simulink model "tether_model"  (R2021b)
settings: Solver=VariableStepAuto  StartTime=0.0  StopTime=1.5*3600  RelTol=1e-3
model workspace (MAT data in the model file):
  At = 7.85398163397e-07
  Is = 1800595238.1
  L = 5000
  a = 7378
  ecc = 0.001
  gamma = 0.00015
  m = 350
  mu_m = 8.22e+22
  p = 0.0031
undefined symbols (not defined in the file): me
settings Model: Creator=woo  LastModifiedBy=woo

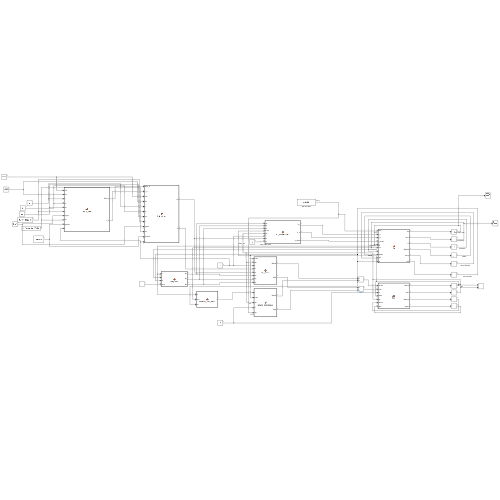
[thumbnail: Simulink's stored preview of the top-level diagram]
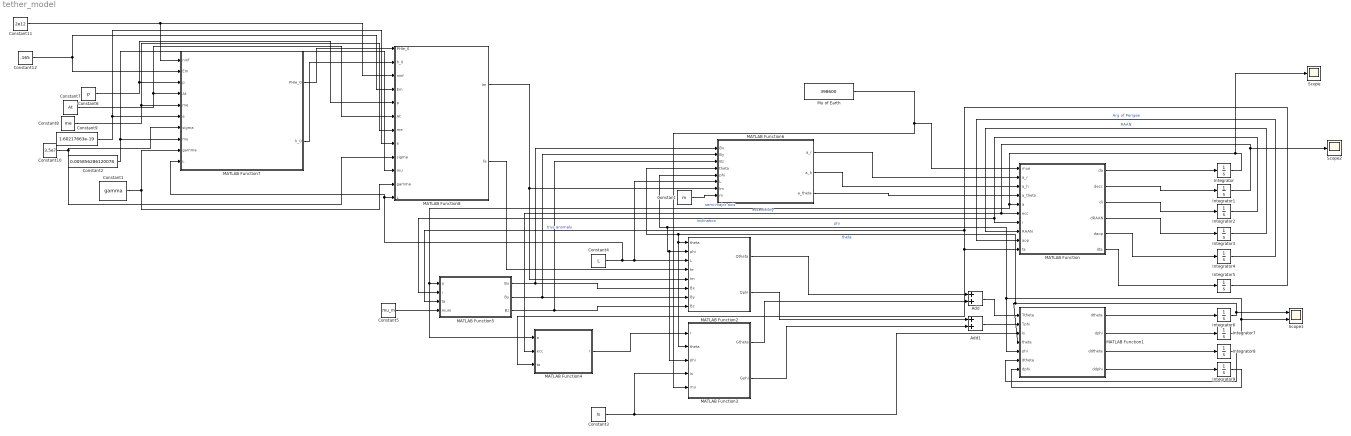
== system tether_model ==
  Add : Sum
  Add1 : Sum
  Constant : Constant  Value=m
  Constant1 : Constant  Value=gamma
  Constant10 : Constant  Value=3.5e7
  Constant11 : Constant  Value=2e12
  Constant12 : Constant  Value=.165
  Constant2 : Constant  Value=0.005856286120078
  Constant3 : Constant  Value=Is
  Constant4 : Constant  Value=L
  Constant5 : Constant  Value=mu_m
  Constant6 : Constant  Value=p
  Constant7 : Constant  Value=At
  Constant8 : Constant  Value=me
  Constant9 : Constant  Value=1.60217663e-19
  Integrator : Integrator  InitialCondition=a
  Integrator1 : Integrator  InitialCondition=ecc
  Integrator2 : Integrator  InitialCondition=deg2rad(25)
  Integrator{3..5,8..9} (5 alike) : Integrator
  Integrator6 : Integrator  InitialCondition=0.1
  Integrator7 : Integrator  InitialCondition=0.1
  MATLAB Function : MATLAB Function  TreatAsAtomicUnit=on
  MATLAB Function1 : MATLAB Function  TreatAsAtomicUnit=on
  MATLAB Function2 : MATLAB Function  TreatAsAtomicUnit=on
  MATLAB Function3 : MATLAB Function  TreatAsAtomicUnit=on
  MATLAB Function4 : MATLAB Function  TreatAsAtomicUnit=on
  MATLAB Function5 : MATLAB Function  TreatAsAtomicUnit=on
  MATLAB Function6 : MATLAB Function  TreatAsAtomicUnit=on
  MATLAB Function7 : MATLAB Function  TreatAsAtomicUnit=on
      settings: RTWSystemCode=Nonreusable function
  MATLAB Function8 : MATLAB Function  TreatAsAtomicUnit=on
  Mu of Earth : Constant  Value=398600  VectorParams1D=off
  Scope : Scope
  Scope1 : Scope  NumInputPorts=2
  Scope2 : Scope
  wires:
  MATLAB Function/1(da) -> Integrator/1
  Integrator/1 -> Scope/1, MATLAB Function4/1(a), MATLAB Function5/1(a), MATLAB Function/5(a)  "semi-major axis"
  MATLAB Function6/3(a_theta) -> MATLAB Function/4(a_theta)
  MATLAB Function6/2(a_h) -> MATLAB Function/3(a_h)
  MATLAB Function6/1(a_r) -> MATLAB Function/2(a_r)
  MATLAB Function/2(decc) -> Integrator1/1
  Integrator1/1 -> Scope2/1, MATLAB Function4/2(ecc), MATLAB Function/6(ecc)  "eccentricity"
  MATLAB Function/3(di) -> Integrator2/1
  Integrator2/1 -> MATLAB Function5/2(i), MATLAB Function/7(i)  "inclination"
  MATLAB Function/4(dRAAN) -> Integrator3/1
  Integrator3/1 -> MATLAB Function/8(RAAN)  "RAAN"
  MATLAB Function/5(daop) -> Integrator4/1
  Integrator4/1 -> MATLAB Function/9(aop)  "Arg of Perigee"
  Integrator5/1 -> MATLAB Function4/3(ta), MATLAB Function/10(ta), MATLAB Function5/3(ta)  "true anomaly"
  MATLAB Function/6(dta) -> Integrator5/1
  Mu of Earth/1 -> MATLAB Function3/5(mu), MATLAB Function/1(mue)
  MATLAB Function1/1(dtheta) -> Integrator6/1
  MATLAB Function1/2(dphi) -> Integrator7/1
  MATLAB Function1/4(ddphi) -> Integrator9/1
  MATLAB Function1/3(ddtheta) -> Integrator8/1
  Integrator9/1 -> MATLAB Function1/7("dphi ")
  Integrator8/1 -> MATLAB Function1/6("dtheta ")
  Integrator7/1 -> MATLAB Function1/5(phi), MATLAB Function3/3(phi), MATLAB Function2/2(phi), MATLAB Function6/5(phi), Scope1/2  "phi"
  Integrator6/1 -> MATLAB Function3/2(theta), MATLAB Function2/1(theta), MATLAB Function6/4(theta), MATLAB Function1/4(theta), Scope1/1  "theta"
  Constant3/1 -> MATLAB Function3/4(Is), MATLAB Function1/3(Is)
  MATLAB Function2/1(Qtheta) -> Add/1
  MATLAB Function3/1(Gtheta) -> Add/2
  Add/1 -> MATLAB Function1/1(Ttheta)
  Add1/1 -> MATLAB Function1/2(Tphi)
  MATLAB Function2/2(Qphi) -> Add1/1
  MATLAB Function3/2(Gphi) -> Add1/2
  Constant4/1 -> MATLAB Function7/10(L), MATLAB Function8/12(L), MATLAB Function6/6(L), MATLAB Function2/3(L)
  MATLAB Function5/1(Bx) -> MATLAB Function6/1(Bx), MATLAB Function2/6(Bx)
  MATLAB Function5/2(By) -> MATLAB Function6/2(By), MATLAB Function2/7(By)
  MATLAB Function5/3(Bz) -> MATLAB Function6/3(Bz), MATLAB Function2/8(Bz)
  Constant5/1 -> MATLAB Function5/4(mum)
  MATLAB Function4/1(r) -> MATLAB Function3/1(r)
  Constant/1 -> MATLAB Function6/8(m)
  MATLAB Function7/1(PHIe_0) -> MATLAB Function8/1(PHIe_0)
  MATLAB Function7/2(h_0) -> MATLAB Function8/2(h_0)
  Constant1/1 -> MATLAB Function7/9(gamma), MATLAB Function8/11(gamma)
  Constant6/1 -> MATLAB Function8/5(p), MATLAB Function7/3(p)
  Constant7/1 -> MATLAB Function8/6(At), MATLAB Function7/4(At)
  Constant2/1 -> MATLAB Function8/10(mu), MATLAB Function7/8(mu)
  Constant8/1 -> MATLAB Function8/7(me), MATLAB Function7/5(me)
  Constant9/1 -> MATLAB Function8/8(e), MATLAB Function7/6(e)
  Constant10/1 -> MATLAB Function8/9(sigma), MATLAB Function7/7(sigma)
  Constant12/1 -> MATLAB Function8/4(Em), MATLAB Function7/2(Em)
  Constant11/1 -> MATLAB Function8/3(ninf), MATLAB Function7/1(ninf)
  MATLAB Function8/1(Im) -> MATLAB Function2/5(Im), MATLAB Function6/7(Im)
  MATLAB Function8/2(fe) -> MATLAB Function2/4(fe)

== matlab function tether_model/MATLAB Function5 ==
  data: a input; Bx output; i input; ta input; mum input; By output; Bz output
function [Bx, By, Bz] = MagField(a, i, ta, mum)
    % Earthrs magnetic field vector in the Orbital Frame of SBET paper
    % SI units output

    % Define variables
    a = COES(1);
    i = COES(3);
    ta = COES(6);
    
%     Bo = 3.12e-5;
%     Bo_over_R3 = Bo/((p/(1+e*cos(ta)))/6378)^3;
    constant = mum/((a*1e3)^3);

    Bx = -2*constant*sin(i)*sin(ta);
    By = -constant*cos(i);
    Bz = constant*sin(i)*cos(ta);

== matlab function tether_model/MATLAB Function6 ==
  data: Bx input; a_r output; By input; Bz input; theta input; phi input; L input; Im input; m input; a_h output; a_theta output
function [a_r, a_h, a_theta] = edt_accelerations(Bx, By, Bz, theta, phi, L, Im, m)
    uhat = [cos(phi)*cos(theta), -sin(phi), cos(phi)*sin(theta)];
    f_orbital = Im*L*cross(uhat, [Bx, By, Bz]);
    a_orbital = f_orbital/m*1e-3'; % force to acceleraction in m to km
    a_r = a_orbital(1);
    a_h = a_orbital(2);
    a_theta = a_orbital(3);

== matlab function tether_model/MATLAB Function7 ==
  data: ninf input; Em input; p input; PHIe_0 output; At input; me input; e input; sigma input; mu input; gamma input; L input; h_0 output
function [PHIe_0, h_0] = solve_bvp(ninf, Em, p, At, me, e, sigma, mu, gamma, L)
    net = load("nna_L4N16_1e2_1e2_100_5km_5mm.mat");
    output = net.net([1;1;1;Em/100;ninf/2e12]);
    PHIe_0 = output(3)*1e5;
    h_0 = output(1)*1e3;
% function [PHIe_0, h_0] = solve_bvp(ninf, Em, p, At, me, e, sigma, mu, gamma, L)
%     parameters = [p, At, me, Em, e, sigma, ninf, mu, gamma];
%     I_B_0 = 1;
%     h0_0 = L/10;
%     s0 = [1;I_B_0;h0_0];
%     opts = optimoptions( 'fsolve' , 'Display' , 'off'  , 'FunctionTolerance' , 1e-8 ,...
%         'StepTolerance' , 1e-8 , 'OptimalityTolerance' , 1e-8 , ...
%         'Algorithm' , 'levenberg-marquardt') ; 
%     [ s0s , F ] = fsolve( @(s)TetherSolveFun(s,parameters,L) , s0 , opts) ;
%     PHIe_0 = s0s(1); 
%     I_B = s0s(2);
%     h_0 = s0s(3);
% 
% 
% end
% 
% 
%     function F = TetherSolveFun(s0, parameters, L) % boundary conditions  
%         p = parameters(1); %perimeter in meters
%         At = parameters(2);
%         me = parameters(3); % mass of electron
%         Em = parameters(4); % Induced electric field; dot(cross(v, B), u)
%         e = parameters(5); % electron charge
%         sigma = parameters(6); % from paper
%         ninf = parameters(7); % ionospheric plasma density 
%         mu = parameters(8); % apparently for atomic oxygen
%         gamma = parameters(9);
%     
%         Ie_0 = 0;
%         PHIe_0 = s0(1); 
%         I_B = s0(2);
%         h0 = s0(3);
%         state0 = [Ie_0, PHIe_0];
%         h_span1 = [0, h0] ;
%         h_span2 = [h0, L] ;
%         opts = odeset( 'RelTol' , 1e-8 , 'AbsTol' , 1e-8 ) ;
%         [t1, s1] = ode45( @bvp_ode_low, h_span1, state0, opts) ;
%         sB = s1(end,:);
%         [t2, s2] = ode45( @bvp_ode_high, h_span2, sB, opts) ;
%         sf = s2(end,:);
%         % [ie, phie]
%     
%         F(1) = sB(1)-I_B; % Ie = max current = I_B, at B
%         F(2) = sB(2); % PHIe = 0 at B
%         F(3) = sf(1)*100; % Ie = 0, I_B, at B
%         F(4) = sum(abs(s1(:,2))-s1(:,2));
%     
%     
%         function dstate = bvp_ode_low(h,state) % equation being solved
%             Ie = state(1);
%             PHIe = state(2);
%               
%             dstate = zeros(2,1);
%             dstate(1) = e*ninf*p/pi*sqrt((2*e/me)*abs(PHIe));
%             dstate(2) = Ie/(sigma*At)-Em;
%         end
%     
%         function dstate = bvp_ode_high(h,state) % equation being solved
%             Ie = state(1);
%             PHIe = state(2);
%         
%             dstate = zeros(2,1);
%             dstate(1) = -e*ninf*p/pi*sqrt((2*e/me)*abs(PHIe))*mu*(1+gamma*abs(PHIe));
%             dstate(2) = Ie/(sigma*At)-Em;
%         end
%     end

== matlab function tether_model/MATLAB Function8 ==
  data: PHIe_0 input; h_0 input; ninf input; Em input; p input; At input; me input; e input; sigma input; mu input; gamma input; L input; Im output; fe output
function [Im, fe] = find_current(PHIe_0, h_0, ninf, Em, p, At, me, e, sigma, mu, gamma, L)
    h_span = [0, L];
    parameters = [p, At, me, Em, e, sigma, ninf, mu, gamma, h_0];
    opts = odeset( 'RelTol' , 1e-8 , 'AbsTol' , 1e-8 ) ;
    [h, s] = ode45( @current_distribution_diffe, h_span, [0, PHIe_0], opts, parameters) ;
    J1 = 0;
    Iint = 0;
    fe_right = 0;
    for ii = 2:length(h)
        J1 = J1 + ((h_G-h(ii))*(s(ii,1))+(h_G-h(ii-1))*(s(ii-1,1)))/2*(h(ii)-h(ii-1));
        Iint = Iint + (s(ii,1)+s(ii-1,1))/2*(h(ii)-h(ii-1));
        fe_right = fe_right + (h(ii)*s(ii,1) + h(ii-1)*s(ii-1,1))/2 * (h(ii)-h(ii-1));
    end
    epsilon = (J1/Is)*mum/mue_si;
    Im = Iint/L;
    fe = fe_right/(L^2*Im);

== matlab function tether_model/MATLAB Function1 ==
  data: dtheta output; dphi output; Ttheta input; ddtheta output; Tphi input; Is input; theta input; phi input; dtheta input; dphi input; ddphi output
function [dtheta, dphi, ddtheta, ddphi] = fcn(Ttheta, Tphi, Is, theta, phi, dtheta, dphi)
    ddtheta = T(2)/Is;
    ddphi = T(3)/Is;

== matlab function tether_model/MATLAB Function ==
  data: mue input; a_r input; da output; a_h input; a_theta input; a input; ecc input; i input; RAAN input; aop input; ta input; decc output; di output; dRAAN output; daop output; dta output
function [da, decc, di, dRAAN, daop, dta]  = VoP(mue, a_r, a_h, a_theta, a, ecc, i, RAAN, aop, ta)
%     a = state(1);
%     ecc = state(2);
%     i = state(3);
%     RAAN = state(4);
%     aop = state(5);
%     ta = state(6);

    p = a*(1-ecc^2);
    h = sqrt(mue*p);
    r = p/(1+ecc*cos(ta));
    n = sqrt(mue/a^3);
    u = aop + ta;

    da = (2/(n*sqrt(1-ecc^2)))*(ecc*sin(ta)*a_r + (p/r)*a_theta);
    decc = (sqrt(1-ecc^2)/(n*a))*(sin(ta)*a_r + ...
        (cos(ta)+(ecc+cos(ta))/(1+ecc*cos(ta)))*a_theta);
    di = (r*cos(u)/(n*a^2*sqrt(1-ecc^2)))*a_h;
    dRAAN = (r*sin(u)/(n*a^2*sqrt(1-ecc^2)*sin(i)))*a_h;
    daop = (sqrt(1-ecc^2)/(n*a*ecc))*(-cos(ta)*a_r + ...
        sin(ta)*(1+r/p)*a_theta) - (r*cot(i)*sin(u)/h)*a_r;
    dta = h/r^2 + (1/(ecc*h))*(p*cos(ta)*a_r - (p+r)*sin(ta)*a_theta);

== matlab function tether_model/MATLAB Function2 ==
  data: theta input; Qtheta output; phi input; L input; fe input; Im input; Bx input; By input; Bz input; Qphi output
function [Qtheta, Qphi] = edt_torque(theta, phi, L, fe, Im, Bx, By, Bz)
    % x is towards zenith
    % y is -h, rotation is in-plane or theta
    % z is along track, rotation is out-of-plane or phi

    Qtheta = fe*Im*L^2*cos(phi)*(sin(phi)*(Bx*cos(theta)+Bz*sin(theta))+By*cos(phi));
    Qphi = -fe*Im*L^2*(Bx*sin(theta)-Bz*cos(theta));

== matlab function tether_model/MATLAB Function3 ==
  data: r input; Gtheta output; theta input; phi input; Is input; mu input; Gphi output
function [Gtheta, Gphi] = gravity_grad_torque(r, theta, phi, Is, mu)
    % Finds the gravity gradient torque effecting the tether
    % x is towards zenith
    % y is -h, rotation is in-plane or theta
    % z is along track, rotation is out-of-plane or phi
    inertia = [0, 0, 0; 0, Is, 0; 0, 0, Is];

    % Dynamics from "Spacecraft Dynamics and Control"
    u1 = [cos(phi)*cos(theta); -sin(phi); cos(phi)*sin(theta)];
    u2 = [-sin(theta); 0; cos(theta)];
    u3 = [-sin(phi)*cos(theta); -cos(phi); -sin(phi)*sin(theta)];
    tether_rotation = [u1, u2, u3];
    rb = tether_rotation*[r;0;0];

    % transform inertia into eci
    rbcross = [0, -rb(3), rb(2);
                rb(3), 0, -rb(1);
                -rb(2), rb(2), 0];
    Tgg = ((3*mu/r^5 * rbcross*inertia*rb));
    Gtheta = Tgg(2);
    Gphi = Tgg(3);

== matlab function tether_model/MATLAB Function4 ==
  data: a input; r output; ecc input; ta input
function r = distance_from_Earth(a, ecc, ta)
    p = a*(1-ecc^2);
    r = p/(1+ecc*cos(ta));
